simulink model "WorkingModel"  (R2023b)
settings: Solver=FixedStepDiscrete  StartTime=0.0  StopTime=param_sim_time  FixedStep=1/fs  MaxStep=1/fs  RelTol=1e-3
undefined symbols (not defined in the file): analyses, fdesignblkfcn, fs, gcbh, param_tot_samples
libraries: dspstat3 x13, SCGAnalysis_SignalGenerationLib x2
(part 6 of 20)

== system WorkingModel/SCG Analysis/Enabled SCG Analysis Subsystem/All Signals Signal Metric Characterization/SCG Systolic 3DMechAxis Signal Metric Characterization ==
  note: Spectral Distribution: S2 (Mid)
  note: Spectral Distribution: S2 (Lo)
  note: Spectral Distribution: S2 (Hi)
  note: Spectral Distribution: S1 (Hi)
  note: Spectral Distribution: S1 (Mid)
  note: Spectral Distribution: S1 (Lo)
  note: Spectral Distribution: Entire Cycle (Hi)
  note: Spectral Distribution: Entire Cycle (Mid)
  note: Spectral Distribution: Entire Cycle (Lo)
  note: Morphological Variability
  note: Var
  note: S2X SNR
  note: S2 SNR
  note: S1X SNR
  note: S1 SNR
  note: S2 P2P Amplitude
  note: S1 P2P Amplitude
  in_ecg_r_pos : Inport
  in_scg_sig : Inport  Port=2
  Average Cycle-to-cycle Morphological Variability Calculator : Subsystem
  Average S1 peak-to-peak Amplitude Calculator : Subsystem
  Average S2 peak-to-peak Amplitude Calculator : Subsystem
  Average Signal-to-Noise Ratio Calculator : Subsystem  mask{s1snr_flag=on, s1xsnr_flag=on, s2snr_flag=on, s2xsnr_flag=on}
      mask prompts: s1snr_flag "S1 SnR"; s1xsnr_flag "S1X SnR (S2 complex is removed)"; s2snr_flag "S2 SnR"; s2xsnr_flag "S2X SnR (S1 complex is removed)"
      mask DialogControl DescGroupVar Prompt: Signal-to-Noise Ratio Characterization
      mask DialogControl DescTextVar Prompt: Block to quantify the signal to noise ratio of the S1 and S2 complexes. Two types of SnRs can be calculated: the normal SnR (which reflects the ease of performing an independent detection of that complex), and the exclusive SnR (which does not cosider the S2 or S1 complex in the case of the S1 and S2 SnRs, respectively).
      mask DialogControl Control2 Prompt: Choose which SnRs to compute:
  Constant : Constant  Value=s1p2p_flag
  Constant1 : Constant  Value=s2p2p_flag
  Constant2 : Constant  Value=snr_flag
  Constant3 : Constant  Value=var_flag
  Constant4 : Constant  Value=morphvar_flag
  Constant5 : Constant  Value=nsd_flag
  Display : Display
  Mux : Mux  Inputs=11
  Spectral Distribution Calculator : Subsystem  mask{entire_cycle=on, s1=on, s2=on, f_band_lo=[7.5 15], f_band_mid=[15 30], f_band_hi=[30 120]}
      mask prompts: entire_cycle "Entire Cycle"; s1 "S1 Complex"; s2 "S2 Complex"; f_band_lo "Frequency Band Low Limits (Hz)"; f_band_mid "Frequency Band Mid Limits (Hz)"; f_band_hi "Frequency Band Hi Limits (Hz)"
      mask DialogControl DescGroupVar Prompt: Spectral Distribution Calculator
      mask DialogControl DescTextVar Prompt: Block to calculate the (normalized) distrubtions of the power spectral densities of: the entire cycle, the S1 complex, and the S2 complex. First select which combination of spectral distrubtions to calculate. Then enter the frequency limits (in Hz) of the three contiguos bins that will define the spectral distribution.
      mask DialogControl ParameterGroupVar_copy Prompt: Spectral Distributions to Calculate
      mask DialogControl Control4 Prompt: Select which spectral distributions to calculate.
      mask DialogControl ParameterGroupVar Prompt: Bin Frequency Bands
      mask DialogControl Control2 Prompt: Enter the frequency limits (in Hz) inside square brackets for three contiguous bins (e.g. [5 10], [10 40], and [40 120]).
  Variance : Subsystem
  out_metrics : Outport
  wires:
  Mux/1 -> out_metrics/1, Display/1
  Constant5/1 -> Spectral Distribution Calculator/Enable
  Constant4/1 -> Average Cycle-to-cycle Morphological Variability Calculator/Enable
  Constant3/1 -> Variance/Enable
  Constant2/1 -> Average Signal-to-Noise Ratio Calculator/Enable
  Constant1/1 -> Average S2 peak-to-peak Amplitude Calculator/Enable
  Constant/1 -> Average S1 peak-to-peak Amplitude Calculator/Enable
  Variance/1(out_scg_signal_var) -> Mux/7
  Spectral Distribution Calculator/2(out_s1_spectral_distribution) -> Mux/10
  Spectral Distribution Calculator/3(out_s2_spectral_distribution) -> Mux/11
  Spectral Distribution Calculator/1(out_entire_cycle_spectral_distribution) -> Mux/9
  Average Cycle-to-cycle Morphological Variability Calculator/1(out_morphological_variability) -> Mux/8
  Average S2 peak-to-peak Amplitude Calculator/1(out_scg_signal_average_s2p2pamp) -> Mux/2
  Average Signal-to-Noise Ratio Calculator/4(out_scg_signal_average_s2Xsnr) -> Mux/6
  Average Signal-to-Noise Ratio Calculator/3(out_scg_signal_average_s2snr) -> Mux/5
  Average Signal-to-Noise Ratio Calculator/1(out_scg_signal_average_s1snr) -> Mux/3
  Average Signal-to-Noise Ratio Calculator/2(out_scg_signal_average_s1Xsnr) -> Mux/4
  in_ecg_r_pos/1 -> Average Signal-to-Noise Ratio Calculator/1(in_r_pos), Average S1 peak-to-peak Amplitude Calculator/1(in_r_pos), Average S2 peak-to-peak Amplitude Calculator/1(in_r_pos), Average Cycle-to-cycle Morphological Variability Calculator/1(in_r_pos), Spectral Distribution Calculator/1(in_r_pos)
  Average S1 peak-to-peak Amplitude Calculator/1(out_average_s1p2pamp) -> Mux/1
  in_scg_sig/1 -> Average Signal-to-Noise Ratio Calculator/2(in_scg_signal), Variance/1(in_scg_signal), Average Cycle-to-cycle Morphological Variability Calculator/2(in_scg_signal), Spectral Distribution Calculator/2(in_scg_signal), Average S1 peak-to-peak Amplitude Calculator/2(in_scg_sig), Average S2 peak-to-peak Amplitude Calculator/2(in_scg_signal)

== system WorkingModel/SCG Analysis/Enabled SCG Analysis Subsystem/All Signals Signal Metric Characterization/SCG Systolic 3DMinS1p2pProjection Signal Metric Characterization ==
  note: S1 P2P Amplitude
  note: S2 P2P Amplitude
  note: S1 SNR
  note: S1X SNR
  note: S2 SNR
  note: S2X SNR
  note: Var
  note: Morphological Variability
  note: Spectral Distribution: Entire Cycle (Lo)
  note: Spectral Distribution: Entire Cycle (Mid)
  note: Spectral Distribution: Entire Cycle (Hi)
  note: Spectral Distribution: S1 (Lo)
  note: Spectral Distribution: S1 (Mid)
  note: Spectral Distribution: S1 (Hi)
  note: Spectral Distribution: S2 (Hi)
  note: Spectral Distribution: S2 (Lo)
  note: Spectral Distribution: S2 (Mid)
  in_ecg_r_pos : Inport
  in_scg_sig : Inport  Port=2
  Average Cycle-to-cycle Morphological Variability Calculator : Subsystem
  Average S1 peak-to-peak Amplitude Calculator : Subsystem
  Average S2 peak-to-peak Amplitude Calculator : Subsystem
  Average Signal-to-Noise Ratio Calculator : Subsystem  mask{s1snr_flag=on, s1xsnr_flag=on, s2snr_flag=on, s2xsnr_flag=on}
      mask prompts: s1snr_flag "S1 SnR"; s1xsnr_flag "S1X SnR (S2 complex is removed)"; s2snr_flag "S2 SnR"; s2xsnr_flag "S2X SnR (S1 complex is removed)"
      mask DialogControl DescGroupVar Prompt: Signal-to-Noise Ratio Characterization
      mask DialogControl DescTextVar Prompt: Block to quantify the signal to noise ratio of the S1 and S2 complexes. Two types of SnRs can be calculated: the normal SnR (which reflects the ease of performing an independent detection of that complex), and the exclusive SnR (which does not cosider the S2 or S1 complex in the case of the S1 and S2 SnRs, respectively).
      mask DialogControl Control2 Prompt: Choose which SnRs to compute:
  Constant : Constant  Value=s1p2p_flag
  Constant1 : Constant  Value=s2p2p_flag
  Constant2 : Constant  Value=snr_flag
  Constant3 : Constant  Value=var_flag
  Constant4 : Constant  Value=morphvar_flag
  Constant5 : Constant  Value=nsd_flag
  Display : Display
  Mux : Mux  Inputs=11
  Spectral Distribution Calculator : Subsystem  mask{entire_cycle=on, s1=on, s2=on, f_band_lo=[7.5 15], f_band_mid=[15 30], f_band_hi=[30 120]}
      mask prompts: entire_cycle "Entire Cycle"; s1 "S1 Complex"; s2 "S2 Complex"; f_band_lo "Frequency Band Low Limits (Hz)"; f_band_mid "Frequency Band Mid Limits (Hz)"; f_band_hi "Frequency Band Hi Limits (Hz)"
      mask DialogControl DescGroupVar Prompt: Spectral Distribution Calculator
      mask DialogControl DescTextVar Prompt: Block to calculate the (normalized) distrubtions of the power spectral densities of: the entire cycle, the S1 complex, and the S2 complex. First select which combination of spectral distrubtions to calculate. Then enter the frequency limits (in Hz) of the three contiguos bins that will define the spectral distribution.
      mask DialogControl ParameterGroupVar_copy Prompt: Spectral Distributions to Calculate
      mask DialogControl Control4 Prompt: Select which spectral distributions to calculate.
      mask DialogControl ParameterGroupVar Prompt: Bin Frequency Bands
      mask DialogControl Control2 Prompt: Enter the frequency limits (in Hz) inside square brackets for three contiguous bins (e.g. [5 10], [10 40], and [40 120]).
  Variance : Subsystem
  out_metrics : Outport
  wires:
  in_scg_sig/1 -> Average S2 peak-to-peak Amplitude Calculator/2(in_scg_signal), Average S1 peak-to-peak Amplitude Calculator/2(in_scg_sig), Spectral Distribution Calculator/2(in_scg_signal), Average Cycle-to-cycle Morphological Variability Calculator/2(in_scg_signal), Variance/1(in_scg_signal), Average Signal-to-Noise Ratio Calculator/2(in_scg_signal)
  Average S1 peak-to-peak Amplitude Calculator/1(out_average_s1p2pamp) -> Mux/1
  in_ecg_r_pos/1 -> Spectral Distribution Calculator/1(in_r_pos), Average Cycle-to-cycle Morphological Variability Calculator/1(in_r_pos), Average S2 peak-to-peak Amplitude Calculator/1(in_r_pos), Average S1 peak-to-peak Amplitude Calculator/1(in_r_pos), Average Signal-to-Noise Ratio Calculator/1(in_r_pos)
  Average Signal-to-Noise Ratio Calculator/2(out_scg_signal_average_s1Xsnr) -> Mux/4
  Average Signal-to-Noise Ratio Calculator/1(out_scg_signal_average_s1snr) -> Mux/3
  Average Signal-to-Noise Ratio Calculator/3(out_scg_signal_average_s2snr) -> Mux/5
  Average Signal-to-Noise Ratio Calculator/4(out_scg_signal_average_s2Xsnr) -> Mux/6
  Average S2 peak-to-peak Amplitude Calculator/1(out_scg_signal_average_s2p2pamp) -> Mux/2
  Average Cycle-to-cycle Morphological Variability Calculator/1(out_morphological_variability) -> Mux/8
  Spectral Distribution Calculator/1(out_entire_cycle_spectral_distribution) -> Mux/9
  Spectral Distribution Calculator/3(out_s2_spectral_distribution) -> Mux/11
  Spectral Distribution Calculator/2(out_s1_spectral_distribution) -> Mux/10
  Variance/1(out_scg_signal_var) -> Mux/7
  Constant/1 -> Average S1 peak-to-peak Amplitude Calculator/Enable
  Constant1/1 -> Average S2 peak-to-peak Amplitude Calculator/Enable
  Constant2/1 -> Average Signal-to-Noise Ratio Calculator/Enable
  Constant3/1 -> Variance/Enable
  Constant4/1 -> Average Cycle-to-cycle Morphological Variability Calculator/Enable
  Constant5/1 -> Spectral Distribution Calculator/Enable
  Mux/1 -> Display/1, out_metrics/1

== system WorkingModel/SCG Analysis/Enabled SCG Analysis Subsystem/All Signals Signal Metric Characterization/SCG X Signal Metric Characterization ==
  note: S1 P2P Amplitude
  note: S2 P2P Amplitude
  note: S1 SNR
  note: S1X SNR
  note: S2 SNR
  note: S2X SNR
  note: Var
  note: Morphological Variability
  note: Spectral Distribution: Entire Cycle (Lo)
  note: Spectral Distribution: Entire Cycle (Mid)
  note: Spectral Distribution: Entire Cycle (Hi)
  note: Spectral Distribution: S1 (Lo)
  note: Spectral Distribution: S1 (Mid)
  note: Spectral Distribution: S1 (Hi)
  note: Spectral Distribution: S2 (Hi)
  note: Spectral Distribution: S2 (Lo)
  note: Spectral Distribution: S2 (Mid)
  in_ecg_r_pos : Inport
  in_scg_sig : Inport  Port=2
  Average Cycle-to-cycle Morphological Variability Calculator : Subsystem
  Average S1 peak-to-peak Amplitude Calculator : Subsystem
  Average S2 peak-to-peak Amplitude Calculator : Subsystem
  Average Signal-to-Noise Ratio Calculator : Subsystem  mask{s1snr_flag=on, s1xsnr_flag=on, s2snr_flag=on, s2xsnr_flag=on}
      mask prompts: s1snr_flag "S1 SnR"; s1xsnr_flag "S1X SnR (S2 complex is removed)"; s2snr_flag "S2 SnR"; s2xsnr_flag "S2X SnR (S1 complex is removed)"
      mask DialogControl DescGroupVar Prompt: Signal-to-Noise Ratio Characterization
      mask DialogControl DescTextVar Prompt: Block to quantify the signal to noise ratio of the S1 and S2 complexes. Two types of SnRs can be calculated: the normal SnR (which reflects the ease of performing an independent detection of that complex), and the exclusive SnR (which does not cosider the S2 or S1 complex in the case of the S1 and S2 SnRs, respectively).
      mask DialogControl Control2 Prompt: Choose which SnRs to compute:
  Constant : Constant  Value=s1p2p_flag
  Constant1 : Constant  Value=s2p2p_flag
  Constant2 : Constant  Value=snr_flag
  Constant3 : Constant  Value=var_flag
  Constant4 : Constant  Value=morphvar_flag
  Constant5 : Constant  Value=nsd_flag
  Display : Display
  Mux : Mux  Inputs=11
  Spectral Distribution Calculator : Subsystem  mask{entire_cycle=on, s1=on, s2=on, f_band_lo=[7.5 15], f_band_mid=[15 30], f_band_hi=[30 120]}
      mask prompts: entire_cycle "Entire Cycle"; s1 "S1 Complex"; s2 "S2 Complex"; f_band_lo "Frequency Band Low Limits (Hz)"; f_band_mid "Frequency Band Mid Limits (Hz)"; f_band_hi "Frequency Band Hi Limits (Hz)"
      mask DialogControl DescGroupVar Prompt: Spectral Distribution Calculator
      mask DialogControl DescTextVar Prompt: Block to calculate the (normalized) distrubtions of the power spectral densities of: the entire cycle, the S1 complex, and the S2 complex. First select which combination of spectral distrubtions to calculate. Then enter the frequency limits (in Hz) of the three contiguos bins that will define the spectral distribution.
      mask DialogControl ParameterGroupVar_copy Prompt: Spectral Distributions to Calculate
      mask DialogControl Control4 Prompt: Select which spectral distributions to calculate.
      mask DialogControl ParameterGroupVar Prompt: Bin Frequency Bands
      mask DialogControl Control2 Prompt: Enter the frequency limits (in Hz) inside square brackets for three contiguous bins (e.g. [5 10], [10 40], and [40 120]).
  Variance : Subsystem
  out_metrics : Outport
  wires:
  in_scg_sig/1 -> Average S2 peak-to-peak Amplitude Calculator/2(in_scg_signal), Average S1 peak-to-peak Amplitude Calculator/2(in_scg_sig), Spectral Distribution Calculator/2(in_scg_signal), Average Cycle-to-cycle Morphological Variability Calculator/2(in_scg_signal), Variance/1(in_scg_signal), Average Signal-to-Noise Ratio Calculator/2(in_scg_signal)
  Average S1 peak-to-peak Amplitude Calculator/1(out_average_s1p2pamp) -> Mux/1
  in_ecg_r_pos/1 -> Spectral Distribution Calculator/1(in_r_pos), Average Cycle-to-cycle Morphological Variability Calculator/1(in_r_pos), Average S2 peak-to-peak Amplitude Calculator/1(in_r_pos), Average S1 peak-to-peak Amplitude Calculator/1(in_r_pos), Average Signal-to-Noise Ratio Calculator/1(in_r_pos)
  Average Signal-to-Noise Ratio Calculator/2(out_scg_signal_average_s1Xsnr) -> Mux/4
  Average Signal-to-Noise Ratio Calculator/1(out_scg_signal_average_s1snr) -> Mux/3
  Average Signal-to-Noise Ratio Calculator/3(out_scg_signal_average_s2snr) -> Mux/5
  Average Signal-to-Noise Ratio Calculator/4(out_scg_signal_average_s2Xsnr) -> Mux/6
  Average S2 peak-to-peak Amplitude Calculator/1(out_scg_signal_average_s2p2pamp) -> Mux/2
  Average Cycle-to-cycle Morphological Variability Calculator/1(out_morphological_variability) -> Mux/8
  Spectral Distribution Calculator/1(out_entire_cycle_spectral_distribution) -> Mux/9
  Spectral Distribution Calculator/3(out_s2_spectral_distribution) -> Mux/11
  Spectral Distribution Calculator/2(out_s1_spectral_distribution) -> Mux/10
  Variance/1(out_scg_signal_var) -> Mux/7
  Constant/1 -> Average S1 peak-to-peak Amplitude Calculator/Enable
  Constant1/1 -> Average S2 peak-to-peak Amplitude Calculator/Enable
  Constant2/1 -> Average Signal-to-Noise Ratio Calculator/Enable
  Constant3/1 -> Variance/Enable
  Constant4/1 -> Average Cycle-to-cycle Morphological Variability Calculator/Enable
  Constant5/1 -> Spectral Distribution Calculator/Enable
  Mux/1 -> Display/1, out_metrics/1

== system WorkingModel/SCG Analysis/Enabled SCG Analysis Subsystem/All Signals Signal Metric Characterization/SCG Y Signal Metric Characterization ==
  note: Spectral Distribution: S2 (Mid)
  note: Spectral Distribution: S2 (Lo)
  note: Spectral Distribution: S2 (Hi)
  note: Spectral Distribution: S1 (Hi)
  note: Spectral Distribution: S1 (Mid)
  note: Spectral Distribution: S1 (Lo)
  note: Spectral Distribution: Entire Cycle (Hi)
  note: Spectral Distribution: Entire Cycle (Mid)
  note: Spectral Distribution: Entire Cycle (Lo)
  note: Morphological Variability
  note: Var
  note: S2X SNR
  note: S2 SNR
  note: S1X SNR
  note: S1 SNR
  note: S2 P2P Amplitude
  note: S1 P2P Amplitude
  in_ecg_r_pos : Inport
  in_scg_sig : Inport  Port=2
  Average Cycle-to-cycle Morphological Variability Calculator : Subsystem
  Average S1 peak-to-peak Amplitude Calculator : Subsystem
  Average S2 peak-to-peak Amplitude Calculator : Subsystem
  Average Signal-to-Noise Ratio Calculator : Subsystem  mask{s1snr_flag=on, s1xsnr_flag=on, s2snr_flag=on, s2xsnr_flag=on}
      mask prompts: s1snr_flag "S1 SnR"; s1xsnr_flag "S1X SnR (S2 complex is removed)"; s2snr_flag "S2 SnR"; s2xsnr_flag "S2X SnR (S1 complex is removed)"
      mask DialogControl DescGroupVar Prompt: Signal-to-Noise Ratio Characterization
      mask DialogControl DescTextVar Prompt: Block to quantify the signal to noise ratio of the S1 and S2 complexes. Two types of SnRs can be calculated: the normal SnR (which reflects the ease of performing an independent detection of that complex), and the exclusive SnR (which does not cosider the S2 or S1 complex in the case of the S1 and S2 SnRs, respectively).
      mask DialogControl Control2 Prompt: Choose which SnRs to compute:
  Constant : Constant  Value=s1p2p_flag
  Constant1 : Constant  Value=s2p2p_flag
  Constant2 : Constant  Value=snr_flag
  Constant3 : Constant  Value=var_flag
  Constant4 : Constant  Value=morphvar_flag
  Constant5 : Constant  Value=nsd_flag
  Display : Display
  Mux : Mux  Inputs=11
  Spectral Distribution Calculator : Subsystem  mask{entire_cycle=on, s1=on, s2=on, f_band_lo=[7.5 15], f_band_mid=[15 30], f_band_hi=[30 120]}
      mask prompts: entire_cycle "Entire Cycle"; s1 "S1 Complex"; s2 "S2 Complex"; f_band_lo "Frequency Band Low Limits (Hz)"; f_band_mid "Frequency Band Mid Limits (Hz)"; f_band_hi "Frequency Band Hi Limits (Hz)"
      mask DialogControl DescGroupVar Prompt: Spectral Distribution Calculator
      mask DialogControl DescTextVar Prompt: Block to calculate the (normalized) distrubtions of the power spectral densities of: the entire cycle, the S1 complex, and the S2 complex. First select which combination of spectral distrubtions to calculate. Then enter the frequency limits (in Hz) of the three contiguos bins that will define the spectral distribution.
      mask DialogControl ParameterGroupVar_copy Prompt: Spectral Distributions to Calculate
      mask DialogControl Control4 Prompt: Select which spectral distributions to calculate.
      mask DialogControl ParameterGroupVar Prompt: Bin Frequency Bands
      mask DialogControl Control2 Prompt: Enter the frequency limits (in Hz) inside square brackets for three contiguous bins (e.g. [5 10], [10 40], and [40 120]).
  Variance : Subsystem
  out_metrics : Outport
  wires:
  Mux/1 -> out_metrics/1, Display/1
  Constant5/1 -> Spectral Distribution Calculator/Enable
  Constant4/1 -> Average Cycle-to-cycle Morphological Variability Calculator/Enable
  Constant3/1 -> Variance/Enable
  Constant2/1 -> Average Signal-to-Noise Ratio Calculator/Enable
  Constant1/1 -> Average S2 peak-to-peak Amplitude Calculator/Enable
  Constant/1 -> Average S1 peak-to-peak Amplitude Calculator/Enable
  Variance/1(out_scg_signal_var) -> Mux/7
  Spectral Distribution Calculator/2(out_s1_spectral_distribution) -> Mux/10
  Spectral Distribution Calculator/3(out_s2_spectral_distribution) -> Mux/11
  Spectral Distribution Calculator/1(out_entire_cycle_spectral_distribution) -> Mux/9
  Average Cycle-to-cycle Morphological Variability Calculator/1(out_morphological_variability) -> Mux/8
  Average S2 peak-to-peak Amplitude Calculator/1(out_scg_signal_average_s2p2pamp) -> Mux/2
  Average Signal-to-Noise Ratio Calculator/4(out_scg_signal_average_s2Xsnr) -> Mux/6
  Average Signal-to-Noise Ratio Calculator/3(out_scg_signal_average_s2snr) -> Mux/5
  Average Signal-to-Noise Ratio Calculator/1(out_scg_signal_average_s1snr) -> Mux/3
  Average Signal-to-Noise Ratio Calculator/2(out_scg_signal_average_s1Xsnr) -> Mux/4
  in_ecg_r_pos/1 -> Average Signal-to-Noise Ratio Calculator/1(in_r_pos), Average S1 peak-to-peak Amplitude Calculator/1(in_r_pos), Average S2 peak-to-peak Amplitude Calculator/1(in_r_pos), Average Cycle-to-cycle Morphological Variability Calculator/1(in_r_pos), Spectral Distribution Calculator/1(in_r_pos)
  Average S1 peak-to-peak Amplitude Calculator/1(out_average_s1p2pamp) -> Mux/1
  in_scg_sig/1 -> Average S1 peak-to-peak Amplitude Calculator/2(in_scg_sig), Average S2 peak-to-peak Amplitude Calculator/2(in_scg_signal), Average Signal-to-Noise Ratio Calculator/2(in_scg_signal), Variance/1(in_scg_signal), Average Cycle-to-cycle Morphological Variability Calculator/2(in_scg_signal), Spectral Distribution Calculator/2(in_scg_signal)

== system WorkingModel/SCG Analysis/Enabled SCG Analysis Subsystem/All Signals Signal Metric Characterization/SCG Z Signal Metric Characterization ==
  note: S1 P2P Amplitude
  note: S2 P2P Amplitude
  note: S1 SNR
  note: S1X SNR
  note: S2 SNR
  note: S2X SNR
  note: Var
  note: Morphological Variability
  note: Spectral Distribution: Entire Cycle (Lo)
  note: Spectral Distribution: Entire Cycle (Mid)
  note: Spectral Distribution: Entire Cycle (Hi)
  note: Spectral Distribution: S1 (Lo)
  note: Spectral Distribution: S1 (Mid)
  note: Spectral Distribution: S1 (Hi)
  note: Spectral Distribution: S2 (Hi)
  note: Spectral Distribution: S2 (Lo)
  note: Spectral Distribution: S2 (Mid)
  in_ecg_r_pos : Inport
  in_scg_sig : Inport  Port=2
  Average Cycle-to-cycle Morphological Variability Calculator : Subsystem
  Average S1 peak-to-peak Amplitude Calculator : Subsystem
  Average S2 peak-to-peak Amplitude Calculator : Subsystem
  Average Signal-to-Noise Ratio Calculator : Subsystem  mask{s1snr_flag=on, s1xsnr_flag=on, s2snr_flag=on, s2xsnr_flag=on}
      mask prompts: s1snr_flag "S1 SnR"; s1xsnr_flag "S1X SnR (S2 complex is removed)"; s2snr_flag "S2 SnR"; s2xsnr_flag "S2X SnR (S1 complex is removed)"
      mask DialogControl DescGroupVar Prompt: Signal-to-Noise Ratio Characterization
      mask DialogControl DescTextVar Prompt: Block to quantify the signal to noise ratio of the S1 and S2 complexes. Two types of SnRs can be calculated: the normal SnR (which reflects the ease of performing an independent detection of that complex), and the exclusive SnR (which does not cosider the S2 or S1 complex in the case of the S1 and S2 SnRs, respectively).
      mask DialogControl Control2 Prompt: Choose which SnRs to compute:
  Constant : Constant  Value=s1p2p_flag
  Constant1 : Constant  Value=s2p2p_flag
  Constant2 : Constant  Value=snr_flag
  Constant3 : Constant  Value=var_flag
  Constant4 : Constant  Value=morphvar_flag
  Constant5 : Constant  Value=nsd_flag
  Display : Display
  Mux : Mux  Inputs=11
  Spectral Distribution Calculator : Subsystem  mask{entire_cycle=on, s1=on, s2=on, f_band_lo=[7.5 15], f_band_mid=[15 30], f_band_hi=[30 120]}
      mask prompts: entire_cycle "Entire Cycle"; s1 "S1 Complex"; s2 "S2 Complex"; f_band_lo "Frequency Band Low Limits (Hz)"; f_band_mid "Frequency Band Mid Limits (Hz)"; f_band_hi "Frequency Band Hi Limits (Hz)"
      mask DialogControl DescGroupVar Prompt: Spectral Distribution Calculator
      mask DialogControl DescTextVar Prompt: Block to calculate the (normalized) distrubtions of the power spectral densities of: the entire cycle, the S1 complex, and the S2 complex. First select which combination of spectral distrubtions to calculate. Then enter the frequency limits (in Hz) of the three contiguos bins that will define the spectral distribution.
      mask DialogControl ParameterGroupVar_copy Prompt: Spectral Distributions to Calculate
      mask DialogControl Control4 Prompt: Select which spectral distributions to calculate.
      mask DialogControl ParameterGroupVar Prompt: Bin Frequency Bands
      mask DialogControl Control2 Prompt: Enter the frequency limits (in Hz) inside square brackets for three contiguous bins (e.g. [5 10], [10 40], and [40 120]).
  Variance : Subsystem
  out_metrics : Outport
  wires:
  in_scg_sig/1 -> Average S2 peak-to-peak Amplitude Calculator/2(in_scg_signal), Average S1 peak-to-peak Amplitude Calculator/2(in_scg_sig), Average Signal-to-Noise Ratio Calculator/2(in_scg_signal), Spectral Distribution Calculator/2(in_scg_signal), Average Cycle-to-cycle Morphological Variability Calculator/2(in_scg_signal), Variance/1(in_scg_signal)
  Average S1 peak-to-peak Amplitude Calculator/1(out_average_s1p2pamp) -> Mux/1
  in_ecg_r_pos/1 -> Spectral Distribution Calculator/1(in_r_pos), Average Cycle-to-cycle Morphological Variability Calculator/1(in_r_pos), Average S2 peak-to-peak Amplitude Calculator/1(in_r_pos), Average S1 peak-to-peak Amplitude Calculator/1(in_r_pos), Average Signal-to-Noise Ratio Calculator/1(in_r_pos)
  Average Signal-to-Noise Ratio Calculator/2(out_scg_signal_average_s1Xsnr) -> Mux/4
  Average Signal-to-Noise Ratio Calculator/1(out_scg_signal_average_s1snr) -> Mux/3
  Average Signal-to-Noise Ratio Calculator/3(out_scg_signal_average_s2snr) -> Mux/5
  Average Signal-to-Noise Ratio Calculator/4(out_scg_signal_average_s2Xsnr) -> Mux/6
  Average S2 peak-to-peak Amplitude Calculator/1(out_scg_signal_average_s2p2pamp) -> Mux/2
  Average Cycle-to-cycle Morphological Variability Calculator/1(out_morphological_variability) -> Mux/8
  Spectral Distribution Calculator/1(out_entire_cycle_spectral_distribution) -> Mux/9
  Spectral Distribution Calculator/3(out_s2_spectral_distribution) -> Mux/11
  Spectral Distribution Calculator/2(out_s1_spectral_distribution) -> Mux/10
  Variance/1(out_scg_signal_var) -> Mux/7
  Constant/1 -> Average S1 peak-to-peak Amplitude Calculator/Enable
  Constant1/1 -> Average S2 peak-to-peak Amplitude Calculator/Enable
  Constant2/1 -> Average Signal-to-Noise Ratio Calculator/Enable
  Constant3/1 -> Variance/Enable
  Constant4/1 -> Average Cycle-to-cycle Morphological Variability Calculator/Enable
  Constant5/1 -> Spectral Distribution Calculator/Enable
  Mux/1 -> Display/1, out_metrics/1

== system WorkingModel/SCG Analysis/Enabled SCG Analysis Subsystem/Signal Generation/2DMod Calculator ==
  in_scg_xyz : Inport
  2DMod Calculator : Subsystem
  Constant : Constant  Value=xyz2Dcombo
  Multiport Switch : MultiPortSwitch  SaturateOnIntegerOverflow=off  InputSameDT=off
  xy Selector : Selector  NumberOfDimensions=2  IndexOptions=Select all,Index vector (dialog)  Indices=[1:min(analyses.ecg.RR)],[1 2]  OutputSizes=1,1
  xz Selector2 : Selector  NumberOfDimensions=2  IndexOptions=Select all,Index vector (dialog)  Indices=[1:min(analyses.ecg.RR)],[1 3]  OutputSizes=1,1
  yz Selector1 : Selector  NumberOfDimensions=2  IndexOptions=Select all,Index vector (dialog)  Indices=[1:min(analyses.ecg.RR)],[2 3]  OutputSizes=1,1
  out_2DMod : Outport  VectorParamsAs1DForOutWhenUnconnected=off
  wires:
  2DMod Calculator/1(2D Modulus) -> out_2DMod/1
  in_scg_xyz/1 -> xz Selector2/1, xy Selector/1, yz Selector1/1
  Constant/1 -> Multiport Switch/1
  Multiport Switch/1 -> 2DMod Calculator/1(2D Components)
  xy Selector/1 -> Multiport Switch/2
  yz Selector1/1 -> Multiport Switch/3
  xz Selector2/1 -> Multiport Switch/4

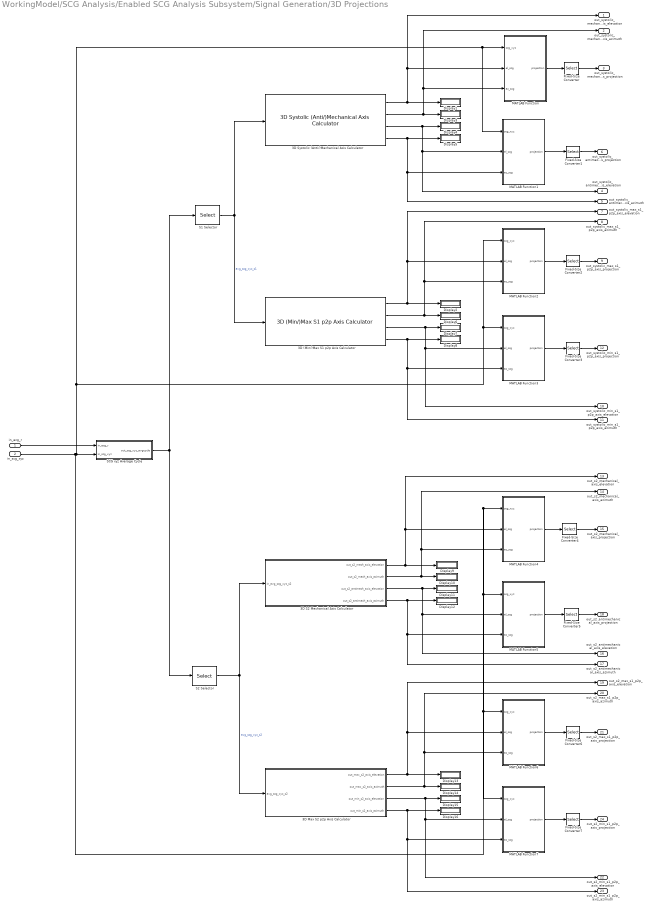
== system WorkingModel/SCG Analysis/Enabled SCG Analysis Subsystem/Signal Generation/3D Projections ==
  in_ecg_r : Inport
  in_scg_xyz : Inport  Port=2
  3D (Min/)Max S1 p2p Axis Calculator : SCGAnalysis_SignalGenerationLib/3D (Min//)Max S1 p2p Axis Calculator  SystemSampleTime=-1  VariantActivationTime=update diagram  AllowFlexibleInterface=on  Latency=0  AutoFrameSizeCalculation=off
      settings: SourceProductName=BioSignal Analysis Library
  3D Max S2 p2p Axis Calculator : Subsystem
      mask Display: image('3D Max S2P2P Axis.png'); % Use "Edit Image" on toolstrip to change.
  3D S2 Mechanical Axis Calculator : Subsystem
      mask Display: image('$imagefile'); % Use "Edit Image" on toolstrip to change.
  3D Systolic (Anti/)Mechanical Axis Calculator : SCGAnalysis_SignalGenerationLib/3D Systolic (Anti//)Mechanical Axis Calculator  SystemSampleTime=-1  VariantActivationTime=update diagram  AllowFlexibleInterface=on  Latency=0  AutoFrameSizeCalculation=off
      settings: SourceProductName=BioSignal Analysis Library
  Display{1..16} (16 alike) : Display
  Fixed-Size Converter{,1..7} (8 alike) : Selector  NumberOfDimensions=2  IndexOptions=Index vector (dialog),Index vector (dialog)  Indices=[1:param_tot_samples],[1]  OutputSizes=1,1
  MATLAB Function : MATLAB Function  TreatAsAtomicUnit=on
  MATLAB Function1 : MATLAB Function  TreatAsAtomicUnit=on
  MATLAB Function2 : MATLAB Function  TreatAsAtomicUnit=on
  MATLAB Function3 : MATLAB Function  TreatAsAtomicUnit=on
  MATLAB Function4 : MATLAB Function  TreatAsAtomicUnit=on
  MATLAB Function5 : MATLAB Function  TreatAsAtomicUnit=on
  MATLAB Function6 : MATLAB Function  TreatAsAtomicUnit=on
  MATLAB Function7 : MATLAB Function  TreatAsAtomicUnit=on
  S1 Selector : Selector  NumberOfDimensions=2  InputPortWidth=3  IndexOptions=Index vector (dialog),Index vector (dialog)  Indices=[1:fs*0.2],[1 2 3]  OutputSizes=1,1
  S2 Selector : Selector  NumberOfDimensions=2  InputPortWidth=3  IndexOptions=Index vector (dialog),Index vector (dialog)  Indices=[fs*0.25:fs*0.5],[1 2 3]  OutputSizes=1,1
  SCG xyz Average Cycle : Subsystem
  out_systolic_mechanical_axis_elevation : Outport
  out_systolic_mechanical_axis_azimuth : Outport  Port=2
  out_systolic_mechanical_axis_projection : Outport  Port=3
  out_systolic_antimechanical_axis_elevation : Outport  Port=4
  out_systolic_antimechanical_axis_azimuth : Outport  Port=5
  out_systolic_antimechanical_axis_projection : Outport  Port=6
  out_systolic_max_s1_p2p_axis_elevation : Outport  Port=7
  out_systolic_max_s1_p2p_axis_azimuth : Outport  Port=8
  out_systolic_max_s1_p2p_axis_projection : Outport  Port=9
  out_systolic_min_s1_p2p_axis_elevation : Outport  Port=10
  out_systolic_min_s1_p2p_axis_azimuth : Outport  Port=11
  out_systolic_min_s1_p2p_axis_projection : Outport  Port=12
  out_s2_mechanical_axis_elevation : Outport  Port=13
  out_s2_mechanical_axis_azimuth : Outport  Port=14
  out_s2_mechanical_axis_projection : Outport  Port=15
  out_s2_antimechanical_axis_elevation : Outport  Port=16
  out_s2_antimechanical_axis_azimuth : Outport  Port=17
  out_s2_antimechanical_axis_projection : Outport  Port=18
  out_s2_max_s1_p2p_axis_elevation : Outport  Port=19
  out_s2_max_s1_p2p_axis_azimuth : Outport  Port=20
  out_s2_max_s1_p2p_axis_projection : Outport  Port=21
  out_s2_min_s1_p2p_axis_elevation : Outport  Port=22
  out_s2_min_s1_p2p_axis_azimuth : Outport  Port=23
  out_s2_min_s1_p2p_axis_projection : Outport  Port=24
  wires:
  S1 Selector/1 -> 3D Systolic (Anti/)Mechanical Axis Calculator/1, 3D (Min/)Max S1 p2p Axis Calculator/1  "avg_scg_xyz_s1"
  SCG xyz Average Cycle/1(out_scg_xyz_avgcycle) -> S1 Selector/1, S2 Selector/1
  MATLAB Function2/1(projection) -> Fixed-Size Converter2/1
  MATLAB Function1/1(projection) -> Fixed-Size Converter1/1
  MATLAB Function/1(projection) -> Fixed-Size Converter/1
  Fixed-Size Converter/1 -> out_systolic_mechanical_axis_projection/1
  Fixed-Size Converter1/1 -> out_systolic_antimechanical_axis_projection/1
  Fixed-Size Converter2/1 -> out_systolic_max_s1_p2p_axis_projection/1
  MATLAB Function3/1(projection) -> Fixed-Size Converter3/1
  Fixed-Size Converter3/1 -> out_systolic_min_s1_p2p_axis_projection/1
  3D Systolic (Anti/)Mechanical Axis Calculator/2 -> Display3/1, out_systolic_mechanical_axis_azimuth/1, MATLAB Function/3(az_scg)
  3D Systolic (Anti/)Mechanical Axis Calculator/3 -> Display4/1, out_systolic_antimechanical_axis_elevation/1, MATLAB Function1/2(el_scg)
  3D Systolic (Anti/)Mechanical Axis Calculator/1 -> Display1/1, out_systolic_mechanical_axis_elevation/1, MATLAB Function/2(el_scg)
  3D Systolic (Anti/)Mechanical Axis Calculator/4 -> Display5/1, out_systolic_antimechanical_axis_azimuth/1, MATLAB Function1/3(az_scg)
  3D (Min/)Max S1 p2p Axis Calculator/4 -> out_systolic_min_s1_p2p_axis_azimuth/1, MATLAB Function3/3(az_scg), Display8/1
  3D (Min/)Max S1 p2p Axis Calculator/2 -> out_systolic_max_s1_p2p_axis_azimuth/1, MATLAB Function2/3(az_scg), Display6/1
  3D (Min/)Max S1 p2p Axis Calculator/3 -> out_systolic_min_s1_p2p_axis_elevation/1, MATLAB Function3/2(el_scg), Display7/1
  3D (Min/)Max S1 p2p Axis Calculator/1 -> out_systolic_max_s1_p2p_axis_elevation/1, MATLAB Function2/2(el_scg), Display2/1
  in_ecg_r/1 -> SCG xyz Average Cycle/1(in_ecg_r)
  S2 Selector/1 -> 3D Max S2 p2p Axis Calculator/1(avg_scg_xyz_s2), 3D S2 Mechanical Axis Calculator/1(in_avg_scg_xyz_s2)  "avg_scg_xyz_s2"
  3D S2 Mechanical Axis Calculator/2(out_s2_mech_axis_azimuth) -> out_s2_mechanical_axis_azimuth/1, MATLAB Function4/3(az_scg), Display10/1
  Fixed-Size Converter4/1 -> out_s2_mechanical_axis_projection/1
  MATLAB Function4/1(projection) -> Fixed-Size Converter4/1
  3D S2 Mechanical Axis Calculator/1(out_s2_mech_axis_elevation) -> out_s2_mechanical_axis_elevation/1, MATLAB Function4/2(el_scg), Display9/1
  3D S2 Mechanical Axis Calculator/3(out_s2_antimech_axis_elevation) -> Display11/1, MATLAB Function5/2(el_scg), out_s2_antimechanical_axis_elevation/1
  Fixed-Size Converter5/1 -> out_s2_antimechanical_axis_projection/1
  MATLAB Function5/1(projection) -> Fixed-Size Converter5/1
  3D S2 Mechanical Axis Calculator/4(out_s2_antimech_axis_azimuth) -> out_s2_antimechanical_axis_azimuth/1, MATLAB Function5/3(az_scg), Display12/1
  Fixed-Size Converter7/1 -> out_s2_min_s1_p2p_axis_projection/1
  3D Max S2 p2p Axis Calculator/1(out_max_s2_axis_elevation) -> out_s2_max_s1_p2p_axis_elevation/1, MATLAB Function6/2(el_scg), Display13/1
  3D Max S2 p2p Axis Calculator/4(out_min_s2_axis_azimuth) -> out_s2_min_s1_p2p_axis_azimuth/1, MATLAB Function7/3(az_scg), Display16/1
  3D Max S2 p2p Axis Calculator/3(out_min_s2_axis_elevation) -> out_s2_min_s1_p2p_axis_elevation/1, MATLAB Function7/2(el_scg), Display15/1
  3D Max S2 p2p Axis Calculator/2(out_max_s2_axis_azimuth) -> out_s2_max_s1_p2p_axis_azimuth/1, MATLAB Function6/3(az_scg), Display14/1
  Fixed-Size Converter6/1 -> out_s2_max_s1_p2p_axis_projection/1
  MATLAB Function6/1(projection) -> Fixed-Size Converter6/1
  MATLAB Function7/1(projection) -> Fixed-Size Converter7/1
  in_scg_xyz/1 -> SCG xyz Average Cycle/2(in_scg_xyz), MATLAB Function2/1(scg_xyz), MATLAB Function3/1(scg_xyz), MATLAB Function/1(scg_xyz), MATLAB Function1/1(scg_xyz), MATLAB Function7/1(scg_xyz), MATLAB Function6/1(scg_xyz), MATLAB Function4/1(scg_xyz), MATLAB Function5/1(scg_xyz)

== system WorkingModel/SCG Analysis/Enabled SCG Analysis Subsystem/Signal Generation/3DMod Calculator ==
  in_scgxyz : Inport
  Square Root1 : Sqrt
  Square1 : Math  Operator=square  SignedPower=on
  Sum1 : Sum  Inputs=+  CollapseMode=Specified dimension  CollapseDim=2
  out_3DMod : Outport  VectorParamsAs1DForOutWhenUnconnected=off
  wires:
  Square1/1 -> Sum1/1
  Sum1/1 -> Square Root1/1
  in_scgxyz/1 -> Square1/1
  Square Root1/1 -> out_3DMod/1

== system WorkingModel/SCG Analysis/Enabled SCG Analysis Subsystem/Systolic Interval Identification/Average Calculator ==
  in_series : Inport
  Average Type : Constant  Value=average_type
  slk_average_calculator : MATLAB Function  TreatAsAtomicUnit=on
  out_average : Outport
  wires:
  in_series/1 -> slk_average_calculator/2(series)
  slk_average_calculator/1(average) -> out_average/1
  Average Type/1 -> slk_average_calculator/1(average_type)

== system WorkingModel/SCG Analysis/Enabled SCG Analysis Subsystem/Systolic Interval Identification/Average Calculator1 ==
  in_series : Inport
  Average Type : Constant  Value=average_type
  slk_average_calculator : MATLAB Function  TreatAsAtomicUnit=on
  out_average : Outport
  wires:
  in_series/1 -> slk_average_calculator/2(series)
  slk_average_calculator/1(average) -> out_average/1
  Average Type/1 -> slk_average_calculator/1(average_type)

== system WorkingModel/SCG Analysis/Enabled SCG Analysis Subsystem/Systolic Interval Identification/Average Calculator2 ==
  in_series : Inport
  Average Type : Constant  Value=average_type
  slk_average_calculator : MATLAB Function  TreatAsAtomicUnit=on
  out_average : Outport
  wires:
  Average Type/1 -> slk_average_calculator/1(average_type)
  slk_average_calculator/1(average) -> out_average/1
  in_series/1 -> slk_average_calculator/2(series)

== system WorkingModel/SCG Analysis/Enabled SCG Analysis Subsystem/Systolic Interval Identification/Average Calculator3 ==
  in_series : Inport
  Average Type : Constant  Value=average_type
  slk_average_calculator : MATLAB Function  TreatAsAtomicUnit=on
  out_average : Outport
  wires:
  in_series/1 -> slk_average_calculator/2(series)
  slk_average_calculator/1(average) -> out_average/1
  Average Type/1 -> slk_average_calculator/1(average_type)

== system WorkingModel/SCG Analysis/Enabled SCG Analysis Subsystem/Systolic Interval Identification/Average Calculator4 ==
  in_series : Inport
  Average Type : Constant  Value=average_type
  slk_average_calculator : MATLAB Function  TreatAsAtomicUnit=on
  out_average : Outport
  wires:
  Average Type/1 -> slk_average_calculator/1(average_type)
  slk_average_calculator/1(average) -> out_average/1
  in_series/1 -> slk_average_calculator/2(series)

== system WorkingModel/SCG Analysis/Enabled SCG Analysis Subsystem/Systolic Interval Identification/Diastolic Fiducial Point Marker ==
  fs : Inport
  in_ecg_r_pos : Inport  Port=2
  in_ecg_t_pos : Inport  Port=3
  in_scg_s2_ref_signal : Inport  Port=4
  in_scg_s2_3DMod : Inport  Port=5
  3D Diastolic Fiducial Point Identifier : MATLAB Function  TreatAsAtomicUnit=on
  Preliminary Diastolic Fiducial Point Identifier : MATLAB Function  TreatAsAtomicUnit=on
  AC : Outport
  MO : Outport  Port=2
  wires:
  3D Diastolic Fiducial Point Identifier/2(MO) -> MO/1
  3D Diastolic Fiducial Point Identifier/1(AC) -> AC/1
  Preliminary Diastolic Fiducial Point Identifier/2(MO_prelim) -> 3D Diastolic Fiducial Point Identifier/3(MO_prelim)
  Preliminary Diastolic Fiducial Point Identifier/1(AC_prelim) -> 3D Diastolic Fiducial Point Identifier/2(AC_prelim)
  in_ecg_r_pos/1 -> Preliminary Diastolic Fiducial Point Identifier/2(ecg_r_pos)
  fs/1 -> 3D Diastolic Fiducial Point Identifier/1(fs), Preliminary Diastolic Fiducial Point Identifier/1(fs)
  in_scg_s2_3DMod/1 -> 3D Diastolic Fiducial Point Identifier/4(scg_s2_3DMod)
  in_ecg_t_pos/1 -> Preliminary Diastolic Fiducial Point Identifier/3(ecg_t_pos)
  in_scg_s2_ref_signal/1 -> Preliminary Diastolic Fiducial Point Identifier/4(scg_s2_ref_signal)

== system WorkingModel/SCG Analysis/Enabled SCG Analysis Subsystem/Systolic Interval Identification/Systolic Fiducial Point Marker ==
  fs : Inport
  in_ecg_r_pos : Inport  Port=2
  in_scg_s1_ref_signal : Inport  Port=3
  in_scg_s1_3DMod : Inport  Port=4
  3D Systolic Fiducial Point Identifier : MATLAB Function  TreatAsAtomicUnit=on
  Preliminary Systolic Fiducial Point Identifier : MATLAB Function  TreatAsAtomicUnit=on
  MC : Outport
  AO : Outport  Port=2
  wires:
  in_scg_s1_ref_signal/1 -> Preliminary Systolic Fiducial Point Identifier/3(scg_s1_ref_signal)
  in_scg_s1_3DMod/1 -> 3D Systolic Fiducial Point Identifier/5(scg_s1_3DMod)
  fs/1 -> Preliminary Systolic Fiducial Point Identifier/1(fs), 3D Systolic Fiducial Point Identifier/1(fs)
  in_ecg_r_pos/1 -> Preliminary Systolic Fiducial Point Identifier/2(ecg_r_pos)
  Preliminary Systolic Fiducial Point Identifier/1(MC_prelim) -> 3D Systolic Fiducial Point Identifier/2(MC_prelim)
  Preliminary Systolic Fiducial Point Identifier/2(IM_prelim) -> 3D Systolic Fiducial Point Identifier/3(IM_prelim)
  Preliminary Systolic Fiducial Point Identifier/3(AO_prelim) -> 3D Systolic Fiducial Point Identifier/4(AO_prelim)
  3D Systolic Fiducial Point Identifier/1(MC) -> MC/1
  3D Systolic Fiducial Point Identifier/2(IM) -> ?
  3D Systolic Fiducial Point Identifier/3(AO) -> AO/1
